simulink model "dec_test"  (R2013b)
settings: Solver=FixedStepDiscrete  SolverMode=SingleTasking  StartTime=0.0  StopTime=100000.0  FixedStep=0.1  RelTol=1e-3
undefined symbols (not defined in the file): pfb_coeff_gen_calc, xlfda_numerator, xlipgetpartsetting
libraries: xbsIndex_r4 x5281, casper_library_misc x30, xps_library x17, dspsigops x16, casper_library_delays x14, xbsReplacements_r4 x2, simulink x1
(part 3 of 62)

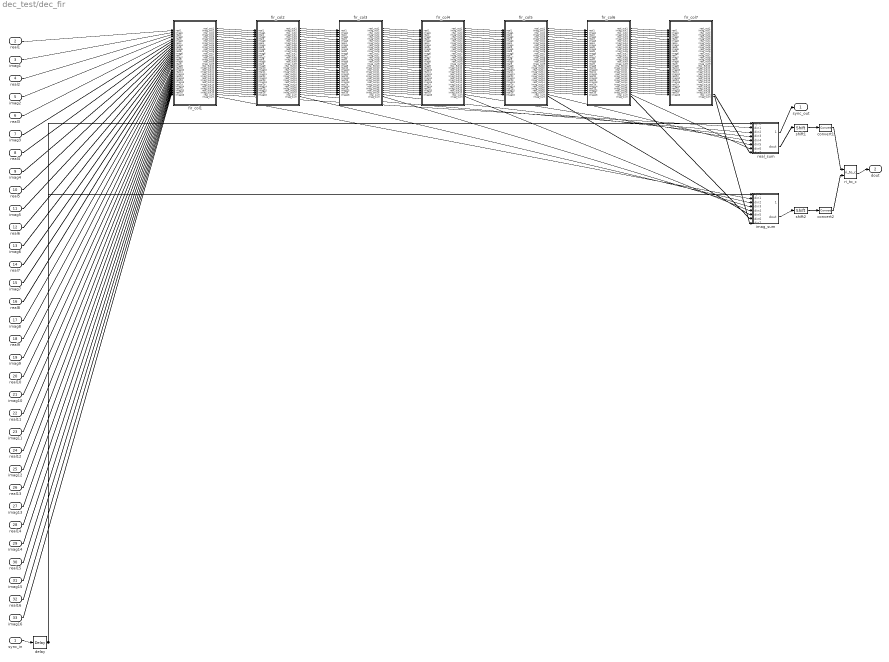
== system dec_test/dec_fir ==
  sync_in : Inport
  real1 : Inport  Port=2
  imag1 : Inport  Port=3
  real2 : Inport  Port=4
  imag2 : Inport  Port=5
  real3 : Inport  Port=6
  imag3 : Inport  Port=7
  real4 : Inport  Port=8
  imag4 : Inport  Port=9
  real5 : Inport  Port=10
  imag5 : Inport  Port=11
  real6 : Inport  Port=12
  imag6 : Inport  Port=13
  real7 : Inport  Port=14
  imag7 : Inport  Port=15
  real8 : Inport  Port=16
  imag8 : Inport  Port=17
  real9 : Inport  Port=18
  imag9 : Inport  Port=19
  real10 : Inport  Port=20
  imag10 : Inport  Port=21
  real11 : Inport  Port=22
  imag11 : Inport  Port=23
  real12 : Inport  Port=24
  imag12 : Inport  Port=25
  real13 : Inport  Port=26
  imag13 : Inport  Port=27
  real14 : Inport  Port=28
  imag14 : Inport  Port=29
  real15 : Inport  Port=30
  imag15 : Inport  Port=31
  real16 : Inport  Port=32
  imag16 : Inport  Port=33
  convert1 : xbsIndex_r4/Convert  gui_display_data_type=Fixed-point  arith_type="Signed  (2's comp)"  n_bits=18  bin_pt=17  float_type=Single  exp_bits=8  fraction_bits=24  quantization="Round  (unbiased: +/- Inf)"  overflow=Wrap  en=off  latency=2  dbl_ovrd=off  pipeline=off  block_type=convert
  convert2 : xbsIndex_r4/Convert  gui_display_data_type=Fixed-point  arith_type="Signed  (2's comp)"  n_bits=18  bin_pt=17  float_type=Single  exp_bits=8  fraction_bits=24  quantization="Round  (unbiased: +/- Inf)"  overflow=Wrap  en=off  latency=2  dbl_ovrd=off  pipeline=off  block_type=convert
  delay : xbsIndex_r4/Delay  rst=off  infoeditControl=Selection of Reset will increase slice count due to use of real FFs and instead of SRLs  en=off  latency=8  dbl_ovrd=off  reg_retiming=off  block_type=delay
  fir_col1 : Subsystem  AncestorBlock=casper_library_downconverter/fir_col  mask(fir_col){n_inputs=16, coeff=[0.0075047   0.0067825   0.0058299   0.0046941   0.0034269   0.0020828  0.00071649 -0.00061865  -0.0018728  -0.0030011  -0.0039654  -0.0047353  -0.0052888   -0.005613  -0.0057043  -0.0055678], add_latency=1, mult_latency=2, coeff_bit_width=25, coeff_bin_pt=24, first_stage_hdl=on, adder_imp=DSP48}
      mask prompts: n_inputs "Inputs"; coeff "Coefficients"; add_latency "Add latency"; mult_latency "Mult Latency"; coeff_bit_width "Coefficient bit width"; coeff_bin_pt "Coefficient binary point"; first_stage_hdl "Implement first stage of adder trees on output as behavioural HDL"; adder_imp "Adder implementation"
      mask init:
      | fir_col_init(gcb, ...
      |     'n_inputs', n_inputs,...
      |     'coeff', coeff, ...
      |     'mult_latency', mult_latency, ...
      |     'add_latency', add_latency, ...
      |     'coeff_bit_width', coeff_bit_width, ...
      |     'coeff_bin_pt', coeff_bin_pt, ...
      |     'first_stage_hdl', first_stage_hdl, ...
      |     'adder_imp', adder_imp);
      mask Help: eval('xlWeb(''http://casper.berkeley.edu/wiki/Fir_col'')')
      mask TypeOptions adder_imp: Behavioral | Fabric | DSP48
  fir_col2 : Subsystem  AncestorBlock=casper_library_downconverter/fir_col  mask(fir_col){n_inputs=16, coeff=[-0.012687   -0.011457  -0.0098785  -0.0080348  -0.0060114  -0.0038941  -0.0017664  0.00029298   0.0022126   0.0039299   0.0053934   0.0065632   0.0074122   0.0079261   0.0081037   0.0079558], add_latency=1, mult_latency=2, coeff_bit_width=25, coeff_bin_pt=24, first_stage_hdl=on, adder_imp=DSP48}
      mask prompts: n_inputs "Inputs"; coeff "Coefficients"; add_latency "Add latency"; mult_latency "Mult Latency"; coeff_bit_width "Coefficient bit width"; coeff_bin_pt "Coefficient binary point"; first_stage_hdl "Implement first stage of adder trees on output as behavioural HDL"; adder_imp "Adder implementation"
      mask init: same as dec_test/dec_fir/fir_col1
      mask Help: eval('xlWeb(''http://casper.berkeley.edu/wiki/Fir_col'')')
      mask TypeOptions adder_imp: Behavioral | Fabric | DSP48
  fir_col3 : Subsystem  AncestorBlock=casper_library_downconverter/fir_col  mask(fir_col){n_inputs=16, coeff=[0.037101    0.031646    0.026085    0.020538    0.015123   0.0099512   0.0051231  0.00072775  -0.0031605  -0.0064835  -0.0092001   -0.011287    -0.01274    -0.01357   -0.013806   -0.013493], add_latency=1, mult_latency=2, coeff_bit_width=25, coeff_bin_pt=24, first_stage_hdl=on, adder_imp=DSP48}
      mask prompts: n_inputs "Inputs"; coeff "Coefficients"; add_latency "Add latency"; mult_latency "Mult Latency"; coeff_bit_width "Coefficient bit width"; coeff_bin_pt "Coefficient binary point"; first_stage_hdl "Implement first stage of adder trees on output as behavioural HDL"; adder_imp "Adder implementation"
      mask init: same as dec_test/dec_fir/fir_col1
      mask Help: eval('xlWeb(''http://casper.berkeley.edu/wiki/Fir_col'')')
      mask TypeOptions adder_imp: Behavioral | Fabric | DSP48
  fir_col4 : Subsystem  AncestorBlock=casper_library_downconverter/fir_col  mask(fir_col){n_inputs=16, coeff=[0.042327    0.047206    0.051624    0.055479    0.058679    0.061149     0.06283     0.06368     0.06368     0.06283    0.061149    0.058679    0.055479    0.051624    0.047206    0.042327], add_latency=1, mult_latency=2, coeff_bit_width=25, coeff_bin_pt=24, first_stage_hdl=on, adder_imp=DSP48}
      mask prompts: n_inputs "Inputs"; coeff "Coefficients"; add_latency "Add latency"; mult_latency "Mult Latency"; coeff_bit_width "Coefficient bit width"; coeff_bin_pt "Coefficient binary point"; first_stage_hdl "Implement first stage of adder trees on output as behavioural HDL"; adder_imp "Adder implementation"
      mask init: same as dec_test/dec_fir/fir_col1
      mask Help: eval('xlWeb(''http://casper.berkeley.edu/wiki/Fir_col'')')
      mask TypeOptions adder_imp: Behavioral | Fabric | DSP48
  fir_col5 : Subsystem  AncestorBlock=casper_library_downconverter/fir_col  mask(fir_col){n_inputs=16, coeff=[-0.013493   -0.013806    -0.01357    -0.01274   -0.011287  -0.0092001  -0.0064835  -0.0031605  0.00072775   0.0051231   0.0099512    0.015123    0.020538    0.026085    0.031646    0.037101], add_latency=1, mult_latency=2, coeff_bit_width=25, coeff_bin_pt=24, first_stage_hdl=on, adder_imp=DSP48}
      mask prompts: n_inputs "Inputs"; coeff "Coefficients"; add_latency "Add latency"; mult_latency "Mult Latency"; coeff_bit_width "Coefficient bit width"; coeff_bin_pt "Coefficient binary point"; first_stage_hdl "Implement first stage of adder trees on output as behavioural HDL"; adder_imp "Adder implementation"
      mask init: same as dec_test/dec_fir/fir_col1
      mask Help: eval('xlWeb(''http://casper.berkeley.edu/wiki/Fir_col'')')
      mask TypeOptions adder_imp: Behavioral | Fabric | DSP48
  fir_col6 : Subsystem  AncestorBlock=casper_library_downconverter/fir_col  mask(fir_col){n_inputs=16, coeff=[0.0079558   0.0081037   0.0079261   0.0074122   0.0065632   0.0053934   0.0039299   0.0022126  0.00029298  -0.0017664  -0.0038941  -0.0060114  -0.0080348  -0.0098785   -0.011457   -0.012687], add_latency=1, mult_latency=2, coeff_bit_width=25, coeff_bin_pt=24, first_stage_hdl=on, adder_imp=DSP48}
      mask prompts: n_inputs "Inputs"; coeff "Coefficients"; add_latency "Add latency"; mult_latency "Mult Latency"; coeff_bit_width "Coefficient bit width"; coeff_bin_pt "Coefficient binary point"; first_stage_hdl "Implement first stage of adder trees on output as behavioural HDL"; adder_imp "Adder implementation"
      mask init: same as dec_test/dec_fir/fir_col1
      mask Help: eval('xlWeb(''http://casper.berkeley.edu/wiki/Fir_col'')')
      mask TypeOptions adder_imp: Behavioral | Fabric | DSP48
  fir_col7 : Subsystem  AncestorBlock=casper_library_downconverter/fir_col  mask(fir_col){n_inputs=16, coeff=[-0.0055678  -0.0057043   -0.005613  -0.0052888  -0.0047353  -0.0039654  -0.0030011  -0.0018728 -0.00061865  0.00071649   0.0020828   0.0034269   0.0046941   0.0058299   0.0067825   0.0075047], add_latency=1, mult_latency=2, coeff_bit_width=25, coeff_bin_pt=24, first_stage_hdl=on, adder_imp=DSP48}
      mask prompts: n_inputs "Inputs"; coeff "Coefficients"; add_latency "Add latency"; mult_latency "Mult Latency"; coeff_bit_width "Coefficient bit width"; coeff_bin_pt "Coefficient binary point"; first_stage_hdl "Implement first stage of adder trees on output as behavioural HDL"; adder_imp "Adder implementation"
      mask init: same as dec_test/dec_fir/fir_col1
      mask Help: eval('xlWeb(''http://casper.berkeley.edu/wiki/Fir_col'')')
      mask TypeOptions adder_imp: Behavioral | Fabric | DSP48
  imag_sum : Subsystem  AncestorBlock=casper_library_misc/adder_tree  mask(adder_tree){n_inputs=7, latency=1, adder_imp=DSP48, first_stage_hdl=off}
      mask prompts: n_inputs "Number of Inputs"; latency "Add Latency"; adder_imp "Adder implementation"; first_stage_hdl "Use behavioural HDL for first stage of adders"
      mask help:
      | Sums all inputs using a tree of adds and delays.
      |
      | Number of inputs: The number of inputs to the block to be summed
      | Add latency: The number of clock cycles to perform one addition (affects timing)..
      | Adder implementation: choice of fabric or DSP48E core, or behavioral HDL
      | Use behavioural HDL for first stage of adders: Causes the first stage of adders to be absorbed into DSP blocks if multipliers precede them (Virtex 5). Overrides Adder implementation
      mask init:
      | adder_tree_init(gcb, ...
      |     'n_inputs', n_inputs, ...
      |     'latency', latency, ...
      |     'adder_imp', adder_imp, ...
      |     'first_stage_hdl', first_stage_hdl);
      settings: AttributesFormatString=latency 3
      mask Help: eval('xlWeb(''http://casper.berkeley.edu/wiki/Adder_tree'')')
      mask TypeOptions adder_imp: Behavioral | Fabric | DSP48
  real_sum : Subsystem  AncestorBlock=casper_library_misc/adder_tree  mask(adder_tree){n_inputs=7, latency=1, adder_imp=DSP48, first_stage_hdl=off}
      mask prompts: n_inputs "Number of Inputs"; latency "Add Latency"; adder_imp "Adder implementation"; first_stage_hdl "Use behavioural HDL for first stage of adders"
      mask help:
      | Sums all inputs using a tree of adds and delays.
      |
      | Number of inputs: The number of inputs to the block to be summed
      | Add latency: The number of clock cycles to perform one addition (affects timing)..
      | Adder implementation: choice of fabric or DSP48E core, or behavioral HDL
      | Use behavioural HDL for first stage of adders: Causes the first stage of adders to be absorbed into DSP blocks if multipliers precede them (Virtex 5). Overrides Adder implementation
      mask init:
      | adder_tree_init(gcb, ...
      |     'n_inputs', n_inputs, ...
      |     'latency', latency, ...
      |     'adder_imp', adder_imp, ...
      |     'first_stage_hdl', first_stage_hdl);
      settings: AttributesFormatString=latency 3
      mask Help: eval('xlWeb(''http://casper.berkeley.edu/wiki/Adder_tree'')')
      mask TypeOptions adder_imp: Behavioral | Fabric | DSP48
  ri_to_c : casper_library_misc/ri_to_c
  shift1 : xbsIndex_r4/Shift  shift_dir=Left  shift_bits=-1  en=off  latency=0  precision=Full  arith_type="Signed  (2's comp)"  n_bits=16  bin_pt=14  quantization=Truncate  overflow=Wrap  dbl_ovrd=off  block_type=shift
  shift2 : xbsIndex_r4/Shift  shift_dir=Left  shift_bits=-1  en=off  latency=0  precision=Full  arith_type="Signed  (2's comp)"  n_bits=16  bin_pt=14  quantization=Truncate  overflow=Wrap  dbl_ovrd=off  block_type=shift
  sync_out : Outport
  dout : Outport  Port=2
  wires:
  real1/1 -> fir_col1/1(real1)
  imag1/1 -> fir_col1/2(imag1)
  real2/1 -> fir_col1/3(real2)
  imag2/1 -> fir_col1/4(imag2)
  real3/1 -> fir_col1/5(real3)
  imag3/1 -> fir_col1/6(imag3)
  real4/1 -> fir_col1/7(real4)
  imag4/1 -> fir_col1/8(imag4)
  real5/1 -> fir_col1/9(real5)
  imag5/1 -> fir_col1/10(imag5)
  real6/1 -> fir_col1/11(real6)
  imag6/1 -> fir_col1/12(imag6)
  real7/1 -> fir_col1/13(real7)
  imag7/1 -> fir_col1/14(imag7)
  real8/1 -> fir_col1/15(real8)
  imag8/1 -> fir_col1/16(imag8)
  real9/1 -> fir_col1/17(real9)
  imag9/1 -> fir_col1/18(imag9)
  real10/1 -> fir_col1/19(real10)
  imag10/1 -> fir_col1/20(imag10)
  real11/1 -> fir_col1/21(real11)
  imag11/1 -> fir_col1/22(imag11)
  real12/1 -> fir_col1/23(real12)
  imag12/1 -> fir_col1/24(imag12)
  real13/1 -> fir_col1/25(real13)
  imag13/1 -> fir_col1/26(imag13)
  real14/1 -> fir_col1/27(real14)
  imag14/1 -> fir_col1/28(imag14)
  real15/1 -> fir_col1/29(real15)
  imag15/1 -> fir_col1/30(imag15)
  real16/1 -> fir_col1/31(real16)
  imag16/1 -> fir_col1/32(imag16)
  fir_col1/33(real_sum) -> real_sum/2(din1)
  fir_col1/34(imag_sum) -> imag_sum/2(din1)
  fir_col1/1(real_out1) -> fir_col2/1(real1)
  fir_col1/2(imag_out1) -> fir_col2/2(imag1)
  fir_col1/3(real_out2) -> fir_col2/3(real2)
  fir_col1/4(imag_out2) -> fir_col2/4(imag2)
  fir_col1/5(real_out3) -> fir_col2/5(real3)
  fir_col1/6(imag_out3) -> fir_col2/6(imag3)
  fir_col1/7(real_out4) -> fir_col2/7(real4)
  fir_col1/8(imag_out4) -> fir_col2/8(imag4)
  fir_col1/9(real_out5) -> fir_col2/9(real5)
  fir_col1/10(imag_out5) -> fir_col2/10(imag5)
  fir_col1/11(real_out6) -> fir_col2/11(real6)
  fir_col1/12(imag_out6) -> fir_col2/12(imag6)
  fir_col1/13(real_out7) -> fir_col2/13(real7)
  fir_col1/14(imag_out7) -> fir_col2/14(imag7)
  fir_col1/15(real_out8) -> fir_col2/15(real8)
  fir_col1/16(imag_out8) -> fir_col2/16(imag8)
  fir_col1/17(real_out9) -> fir_col2/17(real9)
  fir_col1/18(imag_out9) -> fir_col2/18(imag9)
  fir_col1/19(real_out10) -> fir_col2/19(real10)
  fir_col1/20(imag_out10) -> fir_col2/20(imag10)
  fir_col1/21(real_out11) -> fir_col2/21(real11)
  fir_col1/22(imag_out11) -> fir_col2/22(imag11)
  fir_col1/23(real_out12) -> fir_col2/23(real12)
  fir_col1/24(imag_out12) -> fir_col2/24(imag12)
  fir_col1/25(real_out13) -> fir_col2/25(real13)
  fir_col1/26(imag_out13) -> fir_col2/26(imag13)
  fir_col1/27(real_out14) -> fir_col2/27(real14)
  fir_col1/28(imag_out14) -> fir_col2/28(imag14)
  fir_col1/29(real_out15) -> fir_col2/29(real15)
  fir_col1/30(imag_out15) -> fir_col2/30(imag15)
  fir_col1/31(real_out16) -> fir_col2/31(real16)
  fir_col1/32(imag_out16) -> fir_col2/32(imag16)
  fir_col2/33(real_sum) -> real_sum/3(din2)
  fir_col2/34(imag_sum) -> imag_sum/3(din2)
  fir_col2/1(real_out1) -> fir_col3/1(real1)
  fir_col2/2(imag_out1) -> fir_col3/2(imag1)
  fir_col2/3(real_out2) -> fir_col3/3(real2)
  fir_col2/4(imag_out2) -> fir_col3/4(imag2)
  fir_col2/5(real_out3) -> fir_col3/5(real3)
  fir_col2/6(imag_out3) -> fir_col3/6(imag3)
  fir_col2/7(real_out4) -> fir_col3/7(real4)
  fir_col2/8(imag_out4) -> fir_col3/8(imag4)
  fir_col2/9(real_out5) -> fir_col3/9(real5)
  fir_col2/10(imag_out5) -> fir_col3/10(imag5)
  fir_col2/11(real_out6) -> fir_col3/11(real6)
  fir_col2/12(imag_out6) -> fir_col3/12(imag6)
  fir_col2/13(real_out7) -> fir_col3/13(real7)
  fir_col2/14(imag_out7) -> fir_col3/14(imag7)
  fir_col2/15(real_out8) -> fir_col3/15(real8)
  fir_col2/16(imag_out8) -> fir_col3/16(imag8)
  fir_col2/17(real_out9) -> fir_col3/17(real9)
  fir_col2/18(imag_out9) -> fir_col3/18(imag9)
  fir_col2/19(real_out10) -> fir_col3/19(real10)
  fir_col2/20(imag_out10) -> fir_col3/20(imag10)
  fir_col2/21(real_out11) -> fir_col3/21(real11)
  fir_col2/22(imag_out11) -> fir_col3/22(imag11)
  fir_col2/23(real_out12) -> fir_col3/23(real12)
  fir_col2/24(imag_out12) -> fir_col3/24(imag12)
  fir_col2/25(real_out13) -> fir_col3/25(real13)
  fir_col2/26(imag_out13) -> fir_col3/26(imag13)
  fir_col2/27(real_out14) -> fir_col3/27(real14)
  fir_col2/28(imag_out14) -> fir_col3/28(imag14)
  fir_col2/29(real_out15) -> fir_col3/29(real15)
  fir_col2/30(imag_out15) -> fir_col3/30(imag15)
  fir_col2/31(real_out16) -> fir_col3/31(real16)
  fir_col2/32(imag_out16) -> fir_col3/32(imag16)
  fir_col3/33(real_sum) -> real_sum/4(din3)
  fir_col3/34(imag_sum) -> imag_sum/4(din3)
  fir_col3/1(real_out1) -> fir_col4/1(real1)
  fir_col3/2(imag_out1) -> fir_col4/2(imag1)
  fir_col3/3(real_out2) -> fir_col4/3(real2)
  fir_col3/4(imag_out2) -> fir_col4/4(imag2)
  fir_col3/5(real_out3) -> fir_col4/5(real3)
  fir_col3/6(imag_out3) -> fir_col4/6(imag3)
  fir_col3/7(real_out4) -> fir_col4/7(real4)
  fir_col3/8(imag_out4) -> fir_col4/8(imag4)
  fir_col3/9(real_out5) -> fir_col4/9(real5)
  fir_col3/10(imag_out5) -> fir_col4/10(imag5)
  fir_col3/11(real_out6) -> fir_col4/11(real6)
  fir_col3/12(imag_out6) -> fir_col4/12(imag6)
  fir_col3/13(real_out7) -> fir_col4/13(real7)
  fir_col3/14(imag_out7) -> fir_col4/14(imag7)
  fir_col3/15(real_out8) -> fir_col4/15(real8)
  fir_col3/16(imag_out8) -> fir_col4/16(imag8)
  fir_col3/17(real_out9) -> fir_col4/17(real9)
  fir_col3/18(imag_out9) -> fir_col4/18(imag9)
  fir_col3/19(real_out10) -> fir_col4/19(real10)
  fir_col3/20(imag_out10) -> fir_col4/20(imag10)
  fir_col3/21(real_out11) -> fir_col4/21(real11)
  fir_col3/22(imag_out11) -> fir_col4/22(imag11)
  fir_col3/23(real_out12) -> fir_col4/23(real12)
  fir_col3/24(imag_out12) -> fir_col4/24(imag12)
  fir_col3/25(real_out13) -> fir_col4/25(real13)
  fir_col3/26(imag_out13) -> fir_col4/26(imag13)
  fir_col3/27(real_out14) -> fir_col4/27(real14)
  fir_col3/28(imag_out14) -> fir_col4/28(imag14)
  fir_col3/29(real_out15) -> fir_col4/29(real15)
  fir_col3/30(imag_out15) -> fir_col4/30(imag15)
  fir_col3/31(real_out16) -> fir_col4/31(real16)
  fir_col3/32(imag_out16) -> fir_col4/32(imag16)
  fir_col4/33(real_sum) -> real_sum/5(din4)
  fir_col4/34(imag_sum) -> imag_sum/5(din4)
  fir_col4/1(real_out1) -> fir_col5/1(real1)
  fir_col4/2(imag_out1) -> fir_col5/2(imag1)
  fir_col4/3(real_out2) -> fir_col5/3(real2)
  fir_col4/4(imag_out2) -> fir_col5/4(imag2)
  fir_col4/5(real_out3) -> fir_col5/5(real3)
  fir_col4/6(imag_out3) -> fir_col5/6(imag3)
  fir_col4/7(real_out4) -> fir_col5/7(real4)
  fir_col4/8(imag_out4) -> fir_col5/8(imag4)
  fir_col4/9(real_out5) -> fir_col5/9(real5)
  fir_col4/10(imag_out5) -> fir_col5/10(imag5)
  fir_col4/11(real_out6) -> fir_col5/11(real6)
  fir_col4/12(imag_out6) -> fir_col5/12(imag6)
  fir_col4/13(real_out7) -> fir_col5/13(real7)
  fir_col4/14(imag_out7) -> fir_col5/14(imag7)
  fir_col4/15(real_out8) -> fir_col5/15(real8)
  fir_col4/16(imag_out8) -> fir_col5/16(imag8)
  fir_col4/17(real_out9) -> fir_col5/17(real9)
  fir_col4/18(imag_out9) -> fir_col5/18(imag9)
  fir_col4/19(real_out10) -> fir_col5/19(real10)
  fir_col4/20(imag_out10) -> fir_col5/20(imag10)
  fir_col4/21(real_out11) -> fir_col5/21(real11)
  fir_col4/22(imag_out11) -> fir_col5/22(imag11)
  fir_col4/23(real_out12) -> fir_col5/23(real12)
  fir_col4/24(imag_out12) -> fir_col5/24(imag12)
  fir_col4/25(real_out13) -> fir_col5/25(real13)
  fir_col4/26(imag_out13) -> fir_col5/26(imag13)
  fir_col4/27(real_out14) -> fir_col5/27(real14)
  fir_col4/28(imag_out14) -> fir_col5/28(imag14)
  fir_col4/29(real_out15) -> fir_col5/29(real15)
  fir_col4/30(imag_out15) -> fir_col5/30(imag15)
  fir_col4/31(real_out16) -> fir_col5/31(real16)
  fir_col4/32(imag_out16) -> fir_col5/32(imag16)
  fir_col5/33(real_sum) -> real_sum/6(din5)
  fir_col5/34(imag_sum) -> imag_sum/6(din5)
  fir_col5/1(real_out1) -> fir_col6/1(real1)
  fir_col5/2(imag_out1) -> fir_col6/2(imag1)
  fir_col5/3(real_out2) -> fir_col6/3(real2)
  fir_col5/4(imag_out2) -> fir_col6/4(imag2)
  fir_col5/5(real_out3) -> fir_col6/5(real3)
  fir_col5/6(imag_out3) -> fir_col6/6(imag3)
  fir_col5/7(real_out4) -> fir_col6/7(real4)
  fir_col5/8(imag_out4) -> fir_col6/8(imag4)
  fir_col5/9(real_out5) -> fir_col6/9(real5)
  fir_col5/10(imag_out5) -> fir_col6/10(imag5)
  fir_col5/11(real_out6) -> fir_col6/11(real6)
  fir_col5/12(imag_out6) -> fir_col6/12(imag6)
  fir_col5/13(real_out7) -> fir_col6/13(real7)
  fir_col5/14(imag_out7) -> fir_col6/14(imag7)
  fir_col5/15(real_out8) -> fir_col6/15(real8)
  fir_col5/16(imag_out8) -> fir_col6/16(imag8)
  fir_col5/17(real_out9) -> fir_col6/17(real9)
  fir_col5/18(imag_out9) -> fir_col6/18(imag9)
  fir_col5/19(real_out10) -> fir_col6/19(real10)
  fir_col5/20(imag_out10) -> fir_col6/20(imag10)
  fir_col5/21(real_out11) -> fir_col6/21(real11)
  fir_col5/22(imag_out11) -> fir_col6/22(imag11)
  fir_col5/23(real_out12) -> fir_col6/23(real12)
  fir_col5/24(imag_out12) -> fir_col6/24(imag12)
  fir_col5/25(real_out13) -> fir_col6/25(real13)
  fir_col5/26(imag_out13) -> fir_col6/26(imag13)
  fir_col5/27(real_out14) -> fir_col6/27(real14)
  fir_col5/28(imag_out14) -> fir_col6/28(imag14)
  fir_col5/29(real_out15) -> fir_col6/29(real15)
  fir_col5/30(imag_out15) -> fir_col6/30(imag15)
  fir_col5/31(real_out16) -> fir_col6/31(real16)
  fir_col5/32(imag_out16) -> fir_col6/32(imag16)
  fir_col6/33(real_sum) -> real_sum/7(din6)
  fir_col6/34(imag_sum) -> imag_sum/7(din6)
  fir_col6/1(real_out1) -> fir_col7/1(real1)
  fir_col6/2(imag_out1) -> fir_col7/2(imag1)
  fir_col6/3(real_out2) -> fir_col7/3(real2)
  fir_col6/4(imag_out2) -> fir_col7/4(imag2)
  fir_col6/5(real_out3) -> fir_col7/5(real3)
  fir_col6/6(imag_out3) -> fir_col7/6(imag3)
  fir_col6/7(real_out4) -> fir_col7/7(real4)
  fir_col6/8(imag_out4) -> fir_col7/8(imag4)
  fir_col6/9(real_out5) -> fir_col7/9(real5)
  fir_col6/10(imag_out5) -> fir_col7/10(imag5)
  fir_col6/11(real_out6) -> fir_col7/11(real6)
  fir_col6/12(imag_out6) -> fir_col7/12(imag6)
  fir_col6/13(real_out7) -> fir_col7/13(real7)
  fir_col6/14(imag_out7) -> fir_col7/14(imag7)
  fir_col6/15(real_out8) -> fir_col7/15(real8)
  fir_col6/16(imag_out8) -> fir_col7/16(imag8)
  fir_col6/17(real_out9) -> fir_col7/17(real9)
  fir_col6/18(imag_out9) -> fir_col7/18(imag9)
  fir_col6/19(real_out10) -> fir_col7/19(real10)
  fir_col6/20(imag_out10) -> fir_col7/20(imag10)
  fir_col6/21(real_out11) -> fir_col7/21(real11)
  fir_col6/22(imag_out11) -> fir_col7/22(imag11)
  fir_col6/23(real_out12) -> fir_col7/23(real12)
  fir_col6/24(imag_out12) -> fir_col7/24(imag12)
  fir_col6/25(real_out13) -> fir_col7/25(real13)
  fir_col6/26(imag_out13) -> fir_col7/26(imag13)
  fir_col6/27(real_out14) -> fir_col7/27(real14)
  fir_col6/28(imag_out14) -> fir_col7/28(imag14)
  fir_col6/29(real_out15) -> fir_col7/29(real15)
  fir_col6/30(imag_out15) -> fir_col7/30(imag15)
  fir_col6/31(real_out16) -> fir_col7/31(real16)
  fir_col6/32(imag_out16) -> fir_col7/32(imag16)
  fir_col7/33(real_sum) -> real_sum/8(din7)
  fir_col7/34(imag_sum) -> imag_sum/8(din7)
  real_sum/2(dout) -> shift1/1
  imag_sum/2(dout) -> shift2/1
  shift1/1 -> convert1/1
  shift2/1 -> convert2/1
  convert1/1 -> ri_to_c/1
  convert2/1 -> ri_to_c/2
  ri_to_c/1 -> dout/1
  sync_in/1 -> delay/1
  delay/1 -> real_sum/1(sync), imag_sum/1(sync)
  real_sum/1(sync_out) -> sync_out/1

== system dec_test/dout0_0 ==
  addr : Inport
  data_in : Inport  Port=2
  we : Inport  Port=3
  calc_add : Subsystem  mask{data_width=64, addr_width=9, sample_rate=sample_rate}
      mask prompts: data_width "data width"; addr_width "address width"; sample_rate "sample rate"
  convert_addr : xbsIndex_r4/Convert  gui_display_data_type=Fixed-point  arith_type=Unsigned  n_bits=addr_width  bin_pt=0  float_type=Single  exp_bits=8  fraction_bits=24  quantization=Truncate  overflow=Wrap  en=off  latency=0  dbl_ovrd=off  pipeline=off  block_type=convert
      settings: xl_area=[0, 0, 0, 0, 0, 0, 0]
  convert_din1 : xbsIndex_r4/Convert  gui_display_data_type=Fixed-point  arith_type=Unsigned  n_bits=64  bin_pt=0  float_type=Single  exp_bits=8  fraction_bits=24  quantization=Truncate  overflow=Wrap  en=off  latency=0  dbl_ovrd=off  pipeline=off  block_type=convert
      settings: xl_area=[0, 0, 0, 0, 0, 0, 0]
  convert_we : xbsIndex_r4/Convert  gui_display_data_type=Fixed-point  arith_type=Unsigned  n_bits=1  bin_pt=0  float_type=Single  exp_bits=8  fraction_bits=24  quantization=Truncate  overflow=Wrap  en=off  latency=0  dbl_ovrd=off  pipeline=off  block_type=convert
      settings: xl_area=[0, 0, 0, 0, 0, 0, 0]
  dec_test_dout0_0_addr : xbsIndex_r4/Gateway Out  inherit_from_input=off  hdl_port=on  timing_constraint=None  locs_specified=off  LOCs={'A5','B9','A9','C1','A3','G6','E9','A6','A7','A8','B8','B1','B3','D9','B5','B4','B6','C2'}  UseAsDAC=off  DACChannel='1'  block_type=gatewayout
      settings: infoedit="Gateway out block.  Converts Xilinx fixed point inputs into ouputs of type Simulink integer, double, or fixed point.<P><P>Hardware notes:  In hardware these blocks become top level output ports or are discarded, depending on how they are configured."  xl_area=[0, 0, 0, 0, 0, 0, 0]  sginterface={'Nallatech'=>{'xdspkit'=>{'non_memory_mapped_port'=>'uprev_Shared_BRAM_addr'}},'Xilinx'=>{'jtaghwcosim'=>{'non_memory_mapped_port'=>'uprev_Shared_BRAM_addr'},'xdspkit'=>{'non_memory_mapped_port'=>'uprev_Shared_BRAM_addr'}}}
  dec_test_dout0_0_data_in : xbsIndex_r4/Gateway Out  inherit_from_input=off  hdl_port=on  timing_constraint=None  locs_specified=off  LOCs={'B21','B22','A22','B23','B19','C19','A20','A21','A23','B24','A24','A25','E18','D18','C18','B18'}  UseAsDAC=off  DACChannel='1'  block_type=gatewayout
      settings: infoedit="Gateway out block.  Converts Xilinx fixed point inputs into ouputs of type Simulink integer, double, or fixed point.<P><P>Hardware notes:  In hardware these blocks become top level output ports or are discarded, depending on how they are configured."  xl_area=[0, 0, 0, 0, 0, 0, 0]  sginterface={'Nallatech'=>{'xdspkit'=>{'non_memory_mapped_port'=>'uprev_Shared_BRAM_data_in'}},'Xilinx'=>{'jtaghwcosim'=>{'non_memory_mapped_port'=>'uprev_Shared_BRAM_data_in'},'xdspkit'=>{'non_memory_mapped_port'=>'uprev_Shared_BRAM_data_in'}}}
  dec_test_dout0_0_data_out : xbsIndex_r4/Gateway In  gui_display_data_type=Fixed-point  arith_type=Unsigned  n_bits=64  bin_pt=0  preci_type=Single  exp_width=8  frac_width=24  quantization=Truncate  overflow=Wrap  period=sample_rate  dbl_ovrd=off  timing_constraint=None  locs_specified=off  LOCs={}  UseAsADC=off  ADCChannel='1'  inherit_from_input=off  hdl_port=on  block_type=gatewayin
      settings: xl_area=[0, 0, 0, 0, 0, 0, 0]
  dec_test_dout0_0_we : xbsIndex_r4/Gateway Out  inherit_from_input=off  hdl_port=on  timing_constraint=None  locs_specified=off  LOCs={'A14'}  UseAsDAC=off  DACChannel='1'  block_type=gatewayout
      settings: infoedit="Gateway out block.  Converts Xilinx fixed point inputs into ouputs of type Simulink integer, double, or fixed point.<P><P>Hardware notes:  In hardware these blocks become top level output ports or are discarded, depending on how they are configured."  xl_area=[0, 0, 0, 0, 0, 0, 0]
  mem : Subsystem
  munge_in : Subsystem  AncestorBlock=casper_library_flow_control/munge  mask(munge){divisions=2, div_size=[32 32], order=[1  0], arith_type_out=Unsigned, bin_pt_out=0}
      mask prompts: divisions "Number of divisions"; div_size "Division size (bits)"; order "Division packing order"; arith_type_out "Output arithmetic type"; bin_pt_out "Output binary point"
      mask help: Splits an input bus into the specified number of divisions and then recombines them in the order specified (most significant division = 0,least = number divisions-1)
      mask init:
      | munge_init(gcb, ...
      |     'divisions', divisions, ...
      |     'div_size', div_size, ...
      |     'order', order, ...
      |     'arith_type_out', arith_type_out, ...
      |     'bin_pt_out', bin_pt_out);
      settings: AttributesFormatString=|
      | split:[32 32]
      | join:[1 0]
      | Unsigned [64,0]
      mask TypeOptions arith_type_out: Unsigned | Signed  (2's comp) | Floating-point
  munge_out : Subsystem  AncestorBlock=casper_library_flow_control/munge  mask(munge){divisions=2, div_size=[32 32], order=[1  0], arith_type_out=Unsigned, bin_pt_out=0}
      mask prompts: divisions "Number of divisions"; div_size "Division size (bits)"; order "Division packing order"; arith_type_out "Output arithmetic type"; bin_pt_out "Output binary point"
      mask help: Splits an input bus into the specified number of divisions and then recombines them in the order specified (most significant division = 0,least = number divisions-1)
      mask init:
      | munge_init(gcb, ...
      |     'divisions', divisions, ...
      |     'div_size', div_size, ...
      |     'order', order, ...
      |     'arith_type_out', arith_type_out, ...
      |     'bin_pt_out', bin_pt_out);
      settings: AttributesFormatString=|
      | split:[32 32]
      | join:[1 0]
      | Unsigned [64,0]
      mask TypeOptions arith_type_out: Unsigned | Signed  (2's comp) | Floating-point
  data_out : Outport
  wires:
  convert_addr/1 -> dec_test_dout0_0_addr/1
  convert_din1/1 -> dec_test_dout0_0_data_in/1
  data_in/1 -> munge_in/1(din)
  calc_add/1(out) -> convert_addr/1
  dec_test_dout0_0_we/1 -> mem/3(In3)
  dec_test_dout0_0_data_in/1 -> mem/2(In2)
  dec_test_dout0_0_addr/1 -> mem/1(In1)
  convert_we/1 -> dec_test_dout0_0_we/1
  dec_test_dout0_0_data_out/1 -> munge_out/1(din)
  mem/1(Out1) -> dec_test_dout0_0_data_out/1
  addr/1 -> calc_add/1(in)
  we/1 -> convert_we/1
  munge_out/1(dout) -> data_out/1
  munge_in/1(dout) -> convert_din1/1

== system dec_test/dout0_1 ==
  addr : Inport
  data_in : Inport  Port=2
  we : Inport  Port=3
  calc_add : Subsystem  mask{data_width=64, addr_width=9, sample_rate=sample_rate}
      mask prompts: data_width "data width"; addr_width "address width"; sample_rate "sample rate"
  convert_addr : xbsIndex_r4/Convert  gui_display_data_type=Fixed-point  arith_type=Unsigned  n_bits=addr_width  bin_pt=0  float_type=Single  exp_bits=8  fraction_bits=24  quantization=Truncate  overflow=Wrap  en=off  latency=0  dbl_ovrd=off  pipeline=off  block_type=convert
      settings: xl_area=[0, 0, 0, 0, 0, 0, 0]
  convert_din1 : xbsIndex_r4/Convert  gui_display_data_type=Fixed-point  arith_type=Unsigned  n_bits=64  bin_pt=0  float_type=Single  exp_bits=8  fraction_bits=24  quantization=Truncate  overflow=Wrap  en=off  latency=0  dbl_ovrd=off  pipeline=off  block_type=convert
      settings: xl_area=[0, 0, 0, 0, 0, 0, 0]
  convert_we : xbsIndex_r4/Convert  gui_display_data_type=Fixed-point  arith_type=Unsigned  n_bits=1  bin_pt=0  float_type=Single  exp_bits=8  fraction_bits=24  quantization=Truncate  overflow=Wrap  en=off  latency=0  dbl_ovrd=off  pipeline=off  block_type=convert
      settings: xl_area=[0, 0, 0, 0, 0, 0, 0]
  dec_test_dout0_1_addr : xbsIndex_r4/Gateway Out  inherit_from_input=off  hdl_port=on  timing_constraint=None  locs_specified=off  LOCs={'A5','B9','A9','C1','A3','G6','E9','A6','A7','A8','B8','B1','B3','D9','B5','B4','B6','C2'}  UseAsDAC=off  DACChannel='1'  block_type=gatewayout
      settings: infoedit="Gateway out block.  Converts Xilinx fixed point inputs into ouputs of type Simulink integer, double, or fixed point.<P><P>Hardware notes:  In hardware these blocks become top level output ports or are discarded, depending on how they are configured."  xl_area=[0, 0, 0, 0, 0, 0, 0]  sginterface={'Nallatech'=>{'xdspkit'=>{'non_memory_mapped_port'=>'uprev_Shared_BRAM_addr'}},'Xilinx'=>{'jtaghwcosim'=>{'non_memory_mapped_port'=>'uprev_Shared_BRAM_addr'},'xdspkit'=>{'non_memory_mapped_port'=>'uprev_Shared_BRAM_addr'}}}
  dec_test_dout0_1_data_in : xbsIndex_r4/Gateway Out  inherit_from_input=off  hdl_port=on  timing_constraint=None  locs_specified=off  LOCs={'B21','B22','A22','B23','B19','C19','A20','A21','A23','B24','A24','A25','E18','D18','C18','B18'}  UseAsDAC=off  DACChannel='1'  block_type=gatewayout
      settings: infoedit="Gateway out block.  Converts Xilinx fixed point inputs into ouputs of type Simulink integer, double, or fixed point.<P><P>Hardware notes:  In hardware these blocks become top level output ports or are discarded, depending on how they are configured."  xl_area=[0, 0, 0, 0, 0, 0, 0]  sginterface={'Nallatech'=>{'xdspkit'=>{'non_memory_mapped_port'=>'uprev_Shared_BRAM_data_in'}},'Xilinx'=>{'jtaghwcosim'=>{'non_memory_mapped_port'=>'uprev_Shared_BRAM_data_in'},'xdspkit'=>{'non_memory_mapped_port'=>'uprev_Shared_BRAM_data_in'}}}
  dec_test_dout0_1_data_out : xbsIndex_r4/Gateway In  gui_display_data_type=Fixed-point  arith_type=Unsigned  n_bits=64  bin_pt=0  preci_type=Single  exp_width=8  frac_width=24  quantization=Truncate  overflow=Wrap  period=sample_rate  dbl_ovrd=off  timing_constraint=None  locs_specified=off  LOCs={}  UseAsADC=off  ADCChannel='1'  inherit_from_input=off  hdl_port=on  block_type=gatewayin
      settings: xl_area=[0, 0, 0, 0, 0, 0, 0]
  dec_test_dout0_1_we : xbsIndex_r4/Gateway Out  inherit_from_input=off  hdl_port=on  timing_constraint=None  locs_specified=off  LOCs={'A14'}  UseAsDAC=off  DACChannel='1'  block_type=gatewayout
      settings: infoedit="Gateway out block.  Converts Xilinx fixed point inputs into ouputs of type Simulink integer, double, or fixed point.<P><P>Hardware notes:  In hardware these blocks become top level output ports or are discarded, depending on how they are configured."  xl_area=[0, 0, 0, 0, 0, 0, 0]
  mem : Subsystem
  munge_in : Subsystem  AncestorBlock=casper_library_flow_control/munge  mask(munge){divisions=2, div_size=[32 32], order=[1  0], arith_type_out=Unsigned, bin_pt_out=0}
      mask prompts: divisions "Number of divisions"; div_size "Division size (bits)"; order "Division packing order"; arith_type_out "Output arithmetic type"; bin_pt_out "Output binary point"
      mask help: Splits an input bus into the specified number of divisions and then recombines them in the order specified (most significant division = 0,least = number divisions-1)
      mask init:
      | munge_init(gcb, ...
      |     'divisions', divisions, ...
      |     'div_size', div_size, ...
      |     'order', order, ...
      |     'arith_type_out', arith_type_out, ...
      |     'bin_pt_out', bin_pt_out);
      settings: AttributesFormatString=|
      | split:[32 32]
      | join:[1 0]
      | Unsigned [64,0]
      mask TypeOptions arith_type_out: Unsigned | Signed  (2's comp) | Floating-point
  munge_out : Subsystem  AncestorBlock=casper_library_flow_control/munge  mask(munge){divisions=2, div_size=[32 32], order=[1  0], arith_type_out=Unsigned, bin_pt_out=0}
      mask prompts: divisions "Number of divisions"; div_size "Division size (bits)"; order "Division packing order"; arith_type_out "Output arithmetic type"; bin_pt_out "Output binary point"
      mask help: Splits an input bus into the specified number of divisions and then recombines them in the order specified (most significant division = 0,least = number divisions-1)
      mask init:
      | munge_init(gcb, ...
      |     'divisions', divisions, ...
      |     'div_size', div_size, ...
      |     'order', order, ...
      |     'arith_type_out', arith_type_out, ...
      |     'bin_pt_out', bin_pt_out);
      settings: AttributesFormatString=|
      | split:[32 32]
      | join:[1 0]
      | Unsigned [64,0]
      mask TypeOptions arith_type_out: Unsigned | Signed  (2's comp) | Floating-point
  data_out : Outport
  wires:
  munge_in/1(dout) -> convert_din1/1
  munge_out/1(dout) -> data_out/1
  we/1 -> convert_we/1
  addr/1 -> calc_add/1(in)
  mem/1(Out1) -> dec_test_dout0_1_data_out/1
  dec_test_dout0_1_data_out/1 -> munge_out/1(din)
  convert_we/1 -> dec_test_dout0_1_we/1
  dec_test_dout0_1_addr/1 -> mem/1(In1)
  dec_test_dout0_1_data_in/1 -> mem/2(In2)
  dec_test_dout0_1_we/1 -> mem/3(In3)
  calc_add/1(out) -> convert_addr/1
  data_in/1 -> munge_in/1(din)
  convert_din1/1 -> dec_test_dout0_1_data_in/1
  convert_addr/1 -> dec_test_dout0_1_addr/1

== system dec_test/fft_biplex_real_4x ==
  sync : Inport
  shift : Inport  Port=2
  pol0_in : Inport  Port=3
  pol1_in : Inport  Port=4
  pol2_in : Inport  Port=5
  pol3_in : Inport  Port=6
  bi_real_unscr_4x : Subsystem  AncestorBlock=casper_library_ffts_internal/bi_real_unscr_4x  mask(bi_real_unscr_4x){n_inputs=1, FFTSize=8, n_bits=18, bin_pt=17, add_latency=add_latency, conv_latency=conv_latency, bram_latency=bram_latency, bram_map=on, bram_delays=on, dsp48_adders=off, async=off}
      mask prompts: n_inputs "Number simultaneous inputs (2*?)"; FFTSize "Size of FFT (2^?):"; n_bits "Sample Bit Width"; bin_pt "Sample binary point"; add_latency "Add Latency"; conv_latency "Convert Latency"; bram_latency "BRAM Latency"; bram_map "Use BlockRAM for Map"; bram_delays "Use BlockRAM for Delays"; dsp48_adders "Use DSP48s for adders"; async "Asynchonrous operation"
      mask help: FFT internal block.
      mask init:
      | bi_real_unscr_4x_init(gcb, ...
      |     'n_inputs', n_inputs, ...
      |     'FFTSize', FFTSize, ...
      |     'n_bits', n_bits, ...
      |     'bin_pt', bin_pt, ...
      |     'add_latency', add_latency, ...
      |     'conv_latency', conv_latency, ...
      |     'bram_latency', bram_latency, ...
      |     'bram_map', bram_map, ...
      |     'bram_delays', bram_delays, ...
      |     'dsp48_adders', dsp48_adders, ...
      |     'async', async);
  biplex_core : Subsystem  AncestorBlock=casper_library_ffts/biplex_core  mask(biplex_core){n_inputs=1, FFTSize=8, input_bit_width=18, bin_pt_in=17, coeff_bit_width=18, add_latency=1, mult_latency=2, bram_latency=2, conv_latency=1, quantization=Round  (unbiased: +/- Inf), overflow=Saturate, delays_bit_limit=8, coeffs_bit_limit=8, coeff_sharing=on, coeff_decimation=on, max_fanout=4, mult_spec=[2 2 2 2 2 2 2 2], bitgrowth=off, max_bits=19, hardcode_shifts=off, shift_schedule=[1 1], dsp48_adders=off, async=off}
      mask prompts: n_inputs "Number inputs (2*?)"; FFTSize "Size of FFT: (2^? pts)"; input_bit_width "Input Bit Width"; bin_pt_in "Input binary point"; coeff_bit_width "Coefficient Bit Width"; add_latency "Add Latency"; mult_latency "Mult Latency"; bram_latency "BRAM Latency"; conv_latency "Convert latency"; quantization "Quantization Behavior"; overflow "Overflow Behavior"; delays_bit_limit "Number bits above which to implent stage's delays in BRAM (2^? bits)"; coeffs_bit_limit "Number bits above which to store stage's coefficients in BRAM (2^? bits)"; coeff_sharing "BRAM sharing in coeff storage"; coeff_decimation "Store a fraction of coeff factors where useful"; max_fanout "Maximum fanout"; mult_spec "Multiplier impl. (0=core, 1=embedded, 2=behavioural) (left=1st stage, or just one value)"; bitgrowth "Bit growth instead of shift"; max_bits "Maximum number of bits"; hardcode_shifts "Hardcode shift schedule"; shift_schedule "Shift schedule"; dsp48_adders "Use DSP48s for adders"; async "Asynchronous operation"
      mask help: FFT internal block.
      mask init:
      | biplex_core_init(gcb, ...
      |     'n_inputs', n_inputs, ...
      |     'FFTSize', FFTSize,...
      |     'input_bit_width', input_bit_width,...
      |     'bin_pt_in', bin_pt_in,...
      |     'coeff_bit_width', coeff_bit_width,...
      |     'async', async, ...
      |     'add_latency', add_latency,...
      |     'mult_latency', mult_latency,...
      |     'bram_latency', bram_latency,...
      |     'conv_latency', conv_latency, ...
      |     'quantization', quantization,...
      |     'overflow', overflow,...
      |     'delays_bit_limit', delays_bit_limit, ...
      |     'coeffs_bit_limit', coeffs_bit_limit, ...
      |     'coeff_sharing', coeff_sharing, ...
      |     'coeff_decimation', coeff_decimation, ...
      |     'max_fanout', max_fanout, ...
      |     'mult_spec', mult_spec, ...
      |     'bitgrowth', bitgrowth, ...
      |     'max_bits', max_bits, ...
      |     'hardcode_shifts', hardcode_shifts, ...
      |     'shift_schedule', shift_schedule, ...
      |     'dsp48_adders', dsp48_adders);
      settings: AttributesFormatString=8 stages
      mask TypeOptions quantization: Truncate | Round  (unbiased: +/- Inf) | Round  (unbiased: Even Values)
      mask TypeOptions overflow: Wrap | Saturate | Error
      mask Callback hardcode_shifts:
      | hardcode_shifts = get_param(gcb, 'hardcode_shifts');
      | set_param_state(gcb, 'shift_schedule', hardcode_shifts);
      mask Callback dsp48_adders: fft_callback_dsp48_adders(gcb);
  even_bussify : Subsystem  AncestorBlock=casper_library_flow_control/bus_create  mask(bus_create){inputNum=1}
      mask prompts: inputNum "Number of inputs:"
      mask init:
      | bus_create_init(gcb,...
      |     'inputNum', inputNum);
  odd_bussify : Subsystem  AncestorBlock=casper_library_flow_control/bus_create  mask(bus_create){inputNum=1}
      mask prompts: inputNum "Number of inputs:"
      mask init:
      | bus_create_init(gcb,...
      |     'inputNum', inputNum);
  pol0_debus : Subsystem  AncestorBlock=casper_library_flow_control/bus_expand  mask(bus_expand){mode=divisions of equal size, outputNum=1, outputWidth=36, outputBinaryPt=0, outputArithmeticType=0, show_format=off, outputToWorkspace=off, variablePrefix=out, outputToModelAsWell=on}
      mask prompts: outputNum "Number of outputs:"; outputWidth "Output width:"; outputBinaryPt "Output binary point position:"; outputArithmeticType "Output arithmetic type (ufix=0, fix=1, bool=2):"; show_format "Print format string?"; outputToWorkspace "Output to workspace?"; variablePrefix "Variable name prefix:"; outputToModelAsWell "Output to model as well?"
      mask help:
      | Expands a 'bus' made using a bus_create or Xilinx
      | concat block.
      | The input will be divided into the specified number
      | of outputs with the specified arithmetic types.
      | Divisions are made from most significant bit.
      mask init:
      | bus_expand_init(gcb,...
      |     'mode', mode, ...
      |     'outputNum', outputNum, ...
      |     'outputWidth', outputWidth, ...
      |     'outputBinaryPt', outputBinaryPt, ...
      |     'outputArithmeticType', outputArithmeticType, ...
      |     'show_format', show_format, ...
      |     'outputToWorkspace', outputToWorkspace, ...
      |     'variablePrefix', variablePrefix, ...
      |     'outputToModelAsWell', outputToModelAsWell);
      settings: AttributesFormatString=1 outputs
      mask TypeOptions mode: divisions of equal size | divisions of arbitrary size
      mask Callback mode: bus_expand_callback();
      mask Callback outputWidth: bus_expand_callback();
      mask Callback outputToWorkspace: bus_expand_callback();
  pol1_debus : Subsystem  AncestorBlock=casper_library_flow_control/bus_expand  mask(bus_expand){mode=divisions of equal size, outputNum=1, outputWidth=36, outputBinaryPt=0, outputArithmeticType=0, show_format=off, outputToWorkspace=off, variablePrefix=out, outputToModelAsWell=on}
      mask prompts: outputNum "Number of outputs:"; outputWidth "Output width:"; outputBinaryPt "Output binary point position:"; outputArithmeticType "Output arithmetic type (ufix=0, fix=1, bool=2):"; show_format "Print format string?"; outputToWorkspace "Output to workspace?"; variablePrefix "Variable name prefix:"; outputToModelAsWell "Output to model as well?"
      mask help:
      | Expands a 'bus' made using a bus_create or Xilinx
      | concat block.
      | The input will be divided into the specified number
      | of outputs with the specified arithmetic types.
      | Divisions are made from most significant bit.
      mask init: same as dec_test/fft_biplex_real_4x/pol0_debus
      settings: AttributesFormatString=1 outputs
      mask TypeOptions mode: divisions of equal size | divisions of arbitrary size
      mask Callback mode: bus_expand_callback();
      mask Callback outputWidth: bus_expand_callback();
      mask Callback outputToWorkspace: bus_expand_callback();
  pol2_debus : Subsystem  AncestorBlock=casper_library_flow_control/bus_expand  mask(bus_expand){mode=divisions of equal size, outputNum=1, outputWidth=36, outputBinaryPt=0, outputArithmeticType=0, show_format=off, outputToWorkspace=off, variablePrefix=out, outputToModelAsWell=on}
      mask prompts: outputNum "Number of outputs:"; outputWidth "Output width:"; outputBinaryPt "Output binary point position:"; outputArithmeticType "Output arithmetic type (ufix=0, fix=1, bool=2):"; show_format "Print format string?"; outputToWorkspace "Output to workspace?"; variablePrefix "Variable name prefix:"; outputToModelAsWell "Output to model as well?"
      mask help:
      | Expands a 'bus' made using a bus_create or Xilinx
      | concat block.
      | The input will be divided into the specified number
      | of outputs with the specified arithmetic types.
      | Divisions are made from most significant bit.
      mask init: same as dec_test/fft_biplex_real_4x/pol0_debus
      settings: AttributesFormatString=1 outputs
      mask TypeOptions mode: divisions of equal size | divisions of arbitrary size
      mask Callback mode: bus_expand_callback();
      mask Callback outputWidth: bus_expand_callback();
      mask Callback outputToWorkspace: bus_expand_callback();
  pol3_debus : Subsystem  AncestorBlock=casper_library_flow_control/bus_expand  mask(bus_expand){mode=divisions of equal size, outputNum=1, outputWidth=36, outputBinaryPt=0, outputArithmeticType=0, show_format=off, outputToWorkspace=off, variablePrefix=out, outputToModelAsWell=on}
      mask prompts: outputNum "Number of outputs:"; outputWidth "Output width:"; outputBinaryPt "Output binary point position:"; outputArithmeticType "Output arithmetic type (ufix=0, fix=1, bool=2):"; show_format "Print format string?"; outputToWorkspace "Output to workspace?"; variablePrefix "Variable name prefix:"; outputToModelAsWell "Output to model as well?"
      mask help:
      | Expands a 'bus' made using a bus_create or Xilinx
      | concat block.
      | The input will be divided into the specified number
      | of outputs with the specified arithmetic types.
      | Divisions are made from most significant bit.
      mask init: same as dec_test/fft_biplex_real_4x/pol0_debus
      settings: AttributesFormatString=1 outputs
      mask TypeOptions mode: divisions of equal size | divisions of arbitrary size
      mask Callback mode: bus_expand_callback();
      mask Callback outputWidth: bus_expand_callback();
      mask Callback outputToWorkspace: bus_expand_callback();
  ri_to_c0 : Subsystem  AncestorBlock=casper_library_misc/ri_to_c  mask(ri_to_c){}
      mask help:
      | Concatenates real and imaginary inputs into a complex output.
      | Useful for simplifying interconnects.
      | See also: Complex to Real-Imag (c_to_ri)
      mask Help: eval('xlWeb(''http://casper.berkeley.edu/wiki/Ri_to_c'')')
  ri_to_c1 : Subsystem  AncestorBlock=casper_library_misc/ri_to_c  mask(ri_to_c){}
      mask help:
      | Concatenates real and imaginary inputs into a complex output.
      | Useful for simplifying interconnects.
      | See also: Complex to Real-Imag (c_to_ri)
      mask Help: eval('xlWeb(''http://casper.berkeley.edu/wiki/Ri_to_c'')')
  sync_out : Outport
  pol0_out : Outport  Port=2
  pol1_out : Outport  Port=3
  pol2_out : Outport  Port=4
  pol3_out : Outport  Port=5
  of : Outport  Port=6
  wires:
  pol0_debus/1(msb_lsb_out1) -> pol0_out/1
  pol0_in/1 -> ri_to_c0/1(re)
  pol1_in/1 -> ri_to_c0/2(im)
  ri_to_c0/1(c) -> even_bussify/1(in1)
  pol1_debus/1(msb_lsb_out1) -> pol1_out/1
  pol2_debus/1(msb_lsb_out1) -> pol2_out/1
  pol2_in/1 -> ri_to_c1/1(re)
  pol3_in/1 -> ri_to_c1/2(im)
  ri_to_c1/1(c) -> odd_bussify/1(in1)
  pol3_debus/1(msb_lsb_out1) -> pol3_out/1
  sync/1 -> biplex_core/1(sync)
  shift/1 -> biplex_core/2(shift)
  even_bussify/1(bus_out) -> biplex_core/3(pol1)
  odd_bussify/1(bus_out) -> biplex_core/4(pol2)
  biplex_core/4(of) -> of/1
  biplex_core/1(sync_out) -> bi_real_unscr_4x/1(sync)
  biplex_core/2(out1) -> bi_real_unscr_4x/2(even)
  biplex_core/3(out2) -> bi_real_unscr_4x/3(odd)
  bi_real_unscr_4x/1(sync_out) -> sync_out/1
  bi_real_unscr_4x/2(pol1_out) -> pol0_debus/1(bus_in)
  bi_real_unscr_4x/3(pol2_out) -> pol1_debus/1(bus_in)
  bi_real_unscr_4x/4(pol3_out) -> pol2_debus/1(bus_in)
  bi_real_unscr_4x/5(pol4_out) -> pol3_debus/1(bus_in)
